simulink model "attitude3d"  (R2019b)
settings: Solver=ode4  StartTime=0.0  StopTime=6530  FixedStep=10  RelTol=1e-3
values from neighbouring files (symbols this model uses):
  P_E =     [P_E.mat]
  P_F =     [P_F.mat]
  P_X =     [P_X.mat]
undefined symbols (not defined in the file or in its folder): P
libraries: vrlib x14, simulink x5, dspstat3 x4, commfilt2 x2
(part 1 of 2)
settings Model: Creator=ggarrett  LastModifiedBy=ggarrett
settings DataIOCC: ExternalInput=x  LoadExternalInput=on  SaveFormat=Array  TimeSaveName=t  OutputSaveName=F
settings HardwareCC: TargetBitPerLong=64  TargetBitPerPointer=64  TargetBitPerSizeT=64  TargetBitPerPtrDiffT=64  TargetLongLongMode=on  TargetIntDivRoundTo=Zero  TargetEndianess=LittleEndian  TargetWordSize=64  TargetHWDeviceType=MATLAB Host  ProdEqTarget=off
settings RTWCC: Description=Rapid Simulation Target  SystemTargetFile=rsim.tlc  TemplateMakefile=rsim_default_tmf  RTWCompilerOptimization=on
settings RSimTargetCC: TargetLangStandard=C99 (ISO)  GeneratePreprocessorConditionals=Use local settings  PreserveStateflowLocalDataDimensions=off

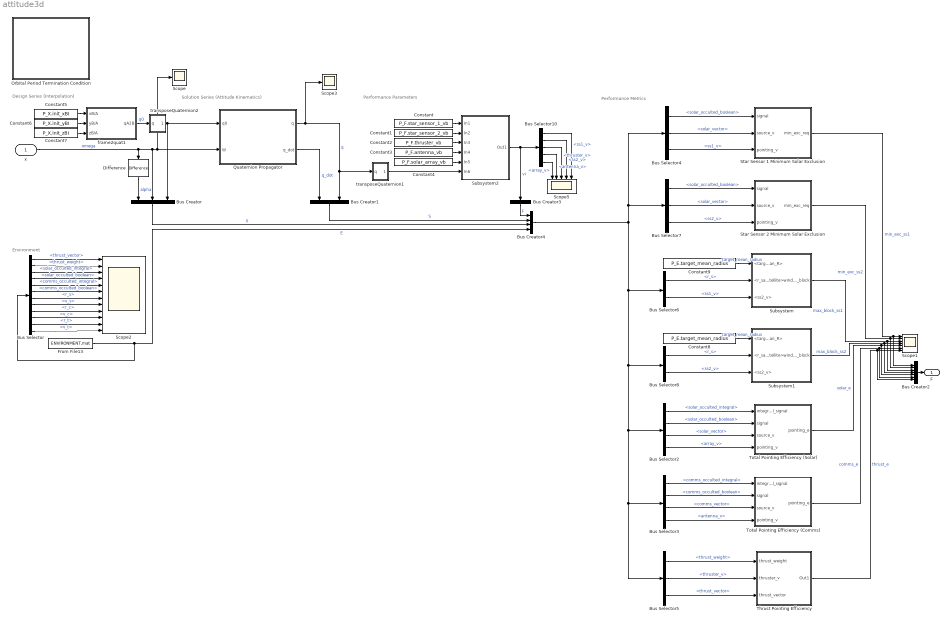
== system attitude3d ==
  note: Performance Metrics
  note: Solution Series (Attitude Kinematics)
  note: Design Series (Interpolation)
  note: Performance Parameters
  note: Environment
  x : Inport  OutDataTypeStr=double  PortDimensions=3
  Bus Creator : BusCreator  Inputs=3
  Bus Creator1 : BusCreator  Inputs=2
  Bus Creator2 : BusCreator  Inputs=7
  Bus Creator3 : BusCreator  Inputs=1
  Bus Creator4 : BusCreator  Inputs=4
  Bus Selector : BusSelector  OutputSignals=thrust_vector,thrust_weight,solar_occulted_integral,solar_occulted_boolean,comms_occulted_integral,comms_occulted_boolean,r_s,v_s,r_c,v_c,r_t,v_t
  Bus Selector10 : BusSelector  OutputSignals=ss1_v,ss2_v,thruster_v,antenna_v,array_v
  Bus Selector2 : BusSelector  OutputSignals=E.solar_occulted_integral,E.solar_occulted_boolean,E.solar_vector,F.vi.array_v
  Bus Selector3 : BusSelector  OutputSignals=E.comms_occulted_integral,E.comms_occulted_boolean,E.comms_vector,F.vi.antenna_v
  Bus Selector4 : BusSelector  OutputSignals=E.solar_occulted_boolean,E.solar_vector,F.vi.ss1_v
  Bus Selector5 : BusSelector  OutputSignals=E.thrust_weight,F.vi.thruster_v,E.thrust_vector
  Bus Selector6 : BusSelector  OutputSignals=E.r_s,F.vi.ss1_v
  Bus Selector7 : BusSelector  OutputSignals=E.solar_occulted_boolean,E.solar_vector,F.vi.ss2_v
  Bus Selector8 : BusSelector  OutputSignals=E.r_s,F.vi.ss2_v
  Constant : Constant  Value=P_F.star_sensor_1_vb
  Constant1 : Constant  Value=P_F.star_sensor_2_vb
  Constant2 : Constant  Value=P_F.thruster_vb
  Constant3 : Constant  Value=P_F.antenna_vb
  Constant4 : Constant  Value=P_F.solar_array_vb
  Constant5 : Constant  Value=P_X.init_xBI
  Constant6 : Constant  Value=P_X.init_yBI
  Constant7 : Constant  Value=P_X.init_zBI
  Constant8 : Constant  Value=P_E.target_mean_radius
  Constant9 : Constant  Value=P_E.target_mean_radius
  Difference : simulink/Discrete/Difference  ICPrevInput=0.0  OutMin=[]  OutMax=[]  OutDataType=fixdt(1, 16)  OutScaling=2^-10  DoSatur=off
  From File13 : FromFile  FileName=ENVIRONMENT.mat  OutDataTypeStr=Bus: ENVIRONMENT  SampleTime=0
  Orbital Period Termination Condition : Subsystem
  Quaternion Propagator : Subsystem
  Scope : Scope
  Scope1 : Scope  NumInputPorts=7
  Scope2 : Scope  NumInputPorts=12
  Scope3 : Scope
  Scope5 : Scope  NumInputPorts=5
  Star Sensor 1 Minimum Solar Exclusion : Subsystem
  Star Sensor 2 Minimum Solar Exclusion : Subsystem
  Subsystem : Subsystem
  Subsystem1 : Subsystem
  Subsystem2 : Subsystem
  Thrust Pointing Efficiency : Subsystem
  Total Pointing Efficiency (Comms) : Subsystem
  Total Pointing Efficiency (Solar) : Subsystem
  frame2quat1 : Subsystem  mask(Compute quaternion from 3 orthogonal unit vectors){Alabel=I, Blabel=B}
      mask prompts: Alabel "Label for origin frame"; Blabel "Label for target frame"
      mask help: Determines the attitude quaternion representing the rotation which transforms the origin frame into the target frame, from the unit vectors of target frame expressed in origin frame.
      mask Display:
      | port_label('input',1,['x',Blabel,'/',Alabel]);
      | port_label('input',2,['y',Blabel,'/',Alabel]);
      | port_label('input',3,['z',Blabel,'/',Alabel]);
      | port_label('output',1,['q',Alabel,'2',Blabel]);
  transposeQuaternion1 : Subsystem  mask(transposeQuaternion){}
      mask help:
      | Compute the transpose (inverse or conjugate) of the input quaternion
      |
      | Inputs:
      |   q     Quaternion
      |
      | Outputs:
      |   qt     Transpose of the input quaternion
      mask Help: eval('starDoc simulink/transposeQuaternion');
      mask Display: disp('q''');
  transposeQuaternion2 : Subsystem  mask(transposeQuaternion){}
      mask help:
      | Compute the transpose (inverse or conjugate) of the input quaternion
      |
      | Inputs:
      |   q     Quaternion
      |
      | Outputs:
      |   qt     Transpose of the input quaternion
      mask Help: eval('starDoc simulink/transposeQuaternion');
      mask Display: disp('q''');
  F : Outport  PortDimensions=7
  wires:
  x/1 -> Bus Creator/2, Scope/1, Quaternion Propagator/2(W), Difference/1  "omega"
  Difference/1 -> Bus Creator/1  "alpha"
  Quaternion Propagator/2(q_dot) -> Bus Creator1/1  "q_dot"
  Bus Creator/1 -> Bus Creator4/3  "X"
  Bus Creator1/1 -> Bus Creator4/2  "S"
  Quaternion Propagator/1(q) -> Scope3/1, Bus Creator1/2, transposeQuaternion1/1(q)  "q"
  Bus Creator3/1 -> Bus Creator4/1  "F"
  Bus Creator4/1 -> Bus Selector5/1, Bus Selector3/1, Bus Selector2/1, Bus Selector8/1, Bus Selector6/1, Bus Selector4/1, Bus Selector7/1
  Bus Selector2/3 -> Total Pointing Efficiency (Solar)/3(source_v)  "<solar_vector>"
  Bus Selector2/4 -> Total Pointing Efficiency (Solar)/4(pointing_v)  "<array_v>"
  Bus Selector2/1 -> Total Pointing Efficiency (Solar)/1(integral_signal)  "<solar_occulted_integral>"
  Bus Selector2/2 -> Total Pointing Efficiency (Solar)/2(signal)  "<solar_occulted_boolean>"
  Bus Selector3/4 -> Total Pointing Efficiency (Comms)/4(pointing_v)  "<antenna_v>"
  Bus Selector3/1 -> Total Pointing Efficiency (Comms)/1(integral_signal)  "<comms_occulted_integral>"
  Bus Selector3/3 -> Total Pointing Efficiency (Comms)/3(source_v)  "<comms_vector>"
  Bus Selector3/2 -> Total Pointing Efficiency (Comms)/2(signal)  "<comms_occulted_boolean>"
  Bus Selector4/3 -> Star Sensor 1 Minimum Solar Exclusion/3(pointing_v)  "<ss1_v>"
  Bus Selector4/1 -> Star Sensor 1 Minimum Solar Exclusion/1(signal)  "<solar_occulted_boolean>"
  Bus Selector4/2 -> Star Sensor 1 Minimum Solar Exclusion/2(source_v)  "<solar_vector>"
  Bus Selector5/3 -> Thrust Pointing Efficiency/3(thrust_vector)  "<thrust_vector>"
  Bus Selector7/3 -> Star Sensor 2 Minimum Solar Exclusion/3(pointing_v)  "<ss2_v>"
  Bus Selector7/1 -> Star Sensor 2 Minimum Solar Exclusion/1(signal)  "<solar_occulted_boolean>"
  Bus Selector7/2 -> Star Sensor 2 Minimum Solar Exclusion/2(source_v)  "<solar_vector>"
  Subsystem1/1(window_block) -> Bus Creator2/4, Scope1/4  "max_block_ss2"
  Subsystem/1(window_block) -> Bus Creator2/3, Scope1/3  "max_block_ss1"
  Star Sensor 2 Minimum Solar Exclusion/1(min_exc_req) -> Bus Creator2/2, Scope1/2  "min_exc_ss2"
  Star Sensor 1 Minimum Solar Exclusion/1(min_exc_req) -> Bus Creator2/1, Scope1/1  "min_exc_ss1"
  Total Pointing Efficiency (Solar)/1(pointing_e) -> Bus Creator2/5, Scope1/5  "solar_e"
  Total Pointing Efficiency (Comms)/1(pointing_e) -> Bus Creator2/6, Scope1/6  "comms_e"
  Thrust Pointing Efficiency/1(Out1) -> Bus Creator2/7, Scope1/7  "thrust_e"
  From File13/1 -> Bus Selector/1, Bus Creator4/4  "E"
  Bus Selector/1 -> Scope2/1  "<thrust_vector>"
  Bus Selector/2 -> Scope2/2  "<thrust_weight>"
  Bus Selector/3 -> Scope2/3  "<solar_occulted_integral>"
  Bus Selector/12 -> Scope2/12  "<v_t>"
  Bus Selector/11 -> Scope2/11  "<r_t>"
  Bus Selector/10 -> Scope2/10  "<v_c>"
  Bus Selector/9 -> Scope2/9  "<r_c>"
  Bus Selector/8 -> Scope2/8  "<v_s>"
  Bus Selector/7 -> Scope2/7  "<r_s>"
  Bus Selector/6 -> Scope2/6  "<comms_occulted_boolean>"
  Bus Selector/5 -> Scope2/5  "<comms_occulted_integral>"
  Bus Selector/4 -> Scope2/4  "<solar_occulted_boolean>"
  Constant5/1 -> frame2quat1/1(xB/A)
  Constant6/1 -> frame2quat1/2(yB/A)
  Bus Selector10/5 -> Scope5/1  "<array_v>"
  Bus Selector10/4 -> Scope5/2  "<antenna_v>"
  Bus Selector10/3 -> Scope5/3  "<thruster_v>"
  Bus Selector10/2 -> Scope5/4  "<ss2_v>"
  Bus Selector10/1 -> Scope5/5  "<ss1_v>"
  Subsystem2/1(Out1) -> Bus Creator3/1, Bus Selector10/1  "vi"
  Constant7/1 -> frame2quat1/3(zB/A)
  Constant/1 -> Subsystem2/1(In1)
  Constant1/1 -> Subsystem2/2(In2)
  Constant2/1 -> Subsystem2/3(In3)
  Constant3/1 -> Subsystem2/4(In4)
  Constant4/1 -> Subsystem2/5(In5)
  transposeQuaternion1/1(q') -> Subsystem2/6(In6)
  Bus Selector8/1 -> Subsystem1/2(<r_satellite>)  "<r_s>"
  Bus Selector8/2 -> Subsystem1/3(<ss2_v>)  "<ss2_v>"
  Constant8/1 -> Subsystem1/1(<target_mean_R>)  "target_mean_radius"
  Bus Selector6/2 -> Subsystem/3(<ss2_v>)  "<ss1_v>"
  Bus Selector6/1 -> Subsystem/2(<r_satellite>)  "<r_s>"
  Constant9/1 -> Subsystem/1(<target_mean_R>)  "target_mean_radius"
  Bus Selector5/1 -> Thrust Pointing Efficiency/1(thrust_weight)  "<thrust_weight>"
  Bus Selector5/2 -> Thrust Pointing Efficiency/2(thruster_v)  "<thruster_v>"
  frame2quat1/1(qA2B) -> transposeQuaternion2/1(q)  "q0"
  transposeQuaternion2/1(q') -> Bus Creator/3, Quaternion Propagator/1(q0)
  Bus Creator2/1 -> F/1

== system attitude3d/Orbital Period Termination Condition ==
  Clock1 : Clock
  Compare To Zero : simulink/Logic and Bit Operations/Compare To Zero  relop=<=  OutDataTypeStr=boolean
  Constant : Constant  Value=0.999*P_E.P
  Scope : Scope  NumInputPorts=2
  Stop Simulation : Stop
  Sum : Sum  Inputs=|-+
  wires:
  Constant/1 -> Scope/1, Sum/2
  Clock1/1 -> Scope/2, Sum/1
  Sum/1 -> Compare To Zero/1
  Compare To Zero/1 -> Stop Simulation/1

== system attitude3d/Quaternion Propagator ==
  q0 : Inport
  W : Inport  Port=2
  Integrator : Integrator  InitialConditionSource=external
  Quaternion Normed : MATLAB Function  TreatAsAtomicUnit=on
  qDot : Subsystem  Tag=40  mask(W2dqdt){}
      mask help:
      | Compute quaternion derivative from instantaneous angular velocity of the rigid body expressed in body frame :
      | dq/dt = 0.5*q*W
      | K. Lagadec 1998
  q : Outport
  q_dot : Outport  Port=2
  wires:
  Integrator/1 -> Quaternion Normed/1(u)
  q0/1 -> Integrator/2
  Quaternion Normed/1(y) -> qDot/1(q), q/1
  W/1 -> qDot/2(W)
  qDot/1(qDot) -> Integrator/1, q_dot/1

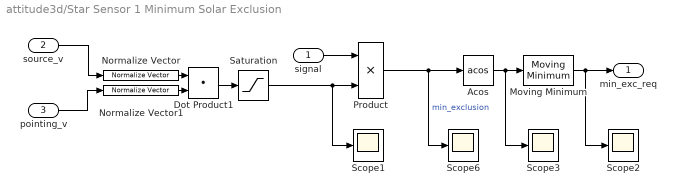
== system attitude3d/Star Sensor 1 Minimum Solar Exclusion ==
  signal : Inport
  source_v : Inport  Port=2
  pointing_v : Inport  Port=3
  Acos : Trigonometry  Operator=acos
  Dot Product1 : DotProduct  InputSameDT=on  OutDataTypeStr=Inherit: Inherit via internal rule
  Moving Minimum : dspstat3/Moving Minimum  SpecifyWindowLength=off  WindowLength=int16(P/10)  SimulateUsing=Code generation
      settings: SourceProductName=DSP System Toolbox  SourceProductBaseCode=DS
  Normalize Vector : vrlib/Utilities/Normalize Vector  maxzero=0
      settings: SourceProductName=Simulink
  Normalize Vector1 : vrlib/Utilities/Normalize Vector  maxzero=0
      settings: SourceProductName=Simulink
  Product : Product
  Saturation : Saturate  UpperLimit=1.0  LowerLimit=0
  Scope{1..3,6} (4 alike) : Scope
  min_exc_req : Outport
  wires:
  Dot Product1/1 -> Saturation/1
  Normalize Vector1/1 -> Dot Product1/2
  signal/1 -> Product/1
  source_v/1 -> Normalize Vector/1
  pointing_v/1 -> Normalize Vector1/1
  Normalize Vector/1 -> Dot Product1/1
  Saturation/1 -> Scope1/1, Product/2
  Product/1 -> Scope6/1, Acos/1  "min_exclusion"
  Acos/1 -> Scope3/1, Moving Minimum/1
  Moving Minimum/1 -> Scope2/1, min_exc_req/1

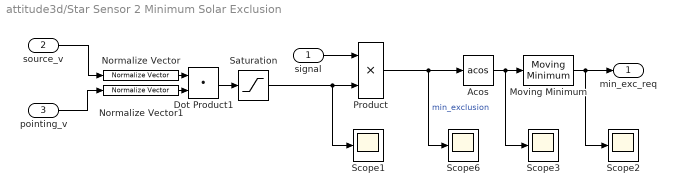
== system attitude3d/Star Sensor 2 Minimum Solar Exclusion ==
  signal : Inport
  source_v : Inport  Port=2
  pointing_v : Inport  Port=3
  Acos : Trigonometry  Operator=acos
  Dot Product1 : DotProduct  InputSameDT=on  OutDataTypeStr=Inherit: Inherit via internal rule
  Moving Minimum : dspstat3/Moving Minimum  SpecifyWindowLength=off  WindowLength=int16(P/10)  SimulateUsing=Code generation
      settings: SourceProductName=DSP System Toolbox  SourceProductBaseCode=DS
  Normalize Vector : vrlib/Utilities/Normalize Vector  maxzero=0
      settings: SourceProductName=Simulink
  Normalize Vector1 : vrlib/Utilities/Normalize Vector  maxzero=0
      settings: SourceProductName=Simulink
  Product : Product
  Saturation : Saturate  UpperLimit=1.0  LowerLimit=0
  Scope{1..3,6} (4 alike) : Scope
  min_exc_req : Outport
  wires:
  Dot Product1/1 -> Saturation/1
  Normalize Vector1/1 -> Dot Product1/2
  signal/1 -> Product/1
  source_v/1 -> Normalize Vector/1
  pointing_v/1 -> Normalize Vector1/1
  Normalize Vector/1 -> Dot Product1/1
  Saturation/1 -> Scope1/1, Product/2
  Product/1 -> Scope6/1, Acos/1  "min_exclusion"
  Acos/1 -> Scope3/1, Moving Minimum/1
  Moving Minimum/1 -> Scope2/1, min_exc_req/1

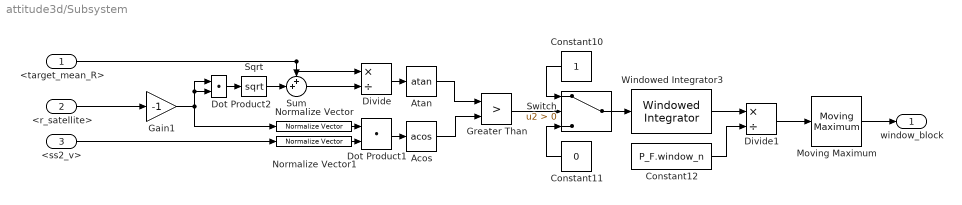
== system attitude3d/Subsystem ==
  <target_mean_R> : Inport
  <r_satellite> : Inport  Port=2
  <ss2_v> : Inport  Port=3
  Acos : Trigonometry  Operator=acos
  Atan : Trigonometry  Operator=atan
  Constant10 : Constant
  Constant11 : Constant  Value=0
  Constant12 : Constant  Value=P_F.window_n
  Divide : Product  Inputs=*/
  Divide1 : Product  Inputs=*/
  Dot Product1 : DotProduct  InputSameDT=on  OutDataTypeStr=Inherit: Inherit via internal rule
  Dot Product2 : DotProduct  InputSameDT=on  OutDataTypeStr=Inherit: Inherit via internal rule
  Gain1 : Gain  Gain=-1
  Greater Than : RelationalOperator  Operator=>  OutDataTypeStr=boolean  RndMeth=Simplest
  Moving Maximum : dspstat3/Moving Maximum  SpecifyWindowLength=off  WindowLength=4  SimulateUsing=Code generation
      settings: SourceProductName=DSP System Toolbox  SourceProductBaseCode=DS
  Normalize Vector : vrlib/Utilities/Normalize Vector  maxzero=0
      settings: SourceProductName=Simulink
  Normalize Vector1 : vrlib/Utilities/Normalize Vector  maxzero=0
      settings: SourceProductName=Simulink
  Sqrt : Sqrt  SaturateOnIntegerOverflow=on
  Sum : Sum  Inputs=++|
  Switch : Switch  Criteria=u2 > Threshold
  Windowed Integrator3 : commfilt2/Windowed Integrator  integperiod=P_F.window_n  InputProcessing=Columns as channels (frame based)  roundingMode=Floor  overflowMode=off  coeffDataTypeStr=Inherit: Same word length as input  coeffMin=[]  coeffMax=[]  coeffLastDataTypeStr=Inherit: Same word length as input  accumDataTypeStr=Inherit: Same as product output  accumLastDataTypeStr=Inherit: Same as product output  outputDataTypeStr=Inherit: Same as accumulator  outputMin=[]  outputMax=[]  outputLastDataTypeStr=Inherit: Same as accumulator
      settings: SourceProductName=Communications Toolbox  SourceProductBaseCode=CM
  window_block : Outport
  wires:
  Sum/1 -> Divide/2
  Dot Product1/1 -> Acos/1
  Normalize Vector/1 -> Dot Product1/1
  Divide1/1 -> Moving Maximum/1
  Constant12/1 -> Divide1/2
  Divide/1 -> Atan/1
  Atan/1 -> Greater Than/1
  Dot Product2/1 -> Sqrt/1
  Moving Maximum/1 -> window_block/1
  Acos/1 -> Greater Than/2
  <r_satellite>/1 -> Gain1/1
  <ss2_v>/1 -> Normalize Vector1/1
  Normalize Vector1/1 -> Dot Product1/2
  Sqrt/1 -> Sum/2
  Constant11/1 -> Switch/3
  Constant10/1 -> Switch/1
  Greater Than/1 -> Switch/2
  <target_mean_R>/1 -> Divide/1, Sum/1
  Gain1/1 -> Normalize Vector/1, Dot Product2/1, Dot Product2/2
  Windowed Integrator3/1 -> Divide1/1
  Switch/1 -> Windowed Integrator3/1

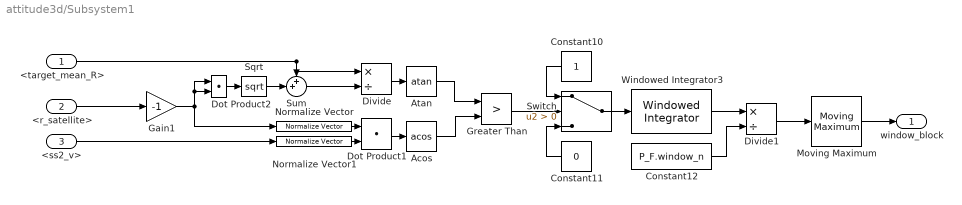
== system attitude3d/Subsystem1 ==
  <target_mean_R> : Inport
  <r_satellite> : Inport  Port=2
  <ss2_v> : Inport  Port=3
  Acos : Trigonometry  Operator=acos
  Atan : Trigonometry  Operator=atan
  Constant10 : Constant
  Constant11 : Constant  Value=0
  Constant12 : Constant  Value=P_F.window_n
  Divide : Product  Inputs=*/
  Divide1 : Product  Inputs=*/
  Dot Product1 : DotProduct  InputSameDT=on  OutDataTypeStr=Inherit: Inherit via internal rule
  Dot Product2 : DotProduct  InputSameDT=on  OutDataTypeStr=Inherit: Inherit via internal rule
  Gain1 : Gain  Gain=-1
  Greater Than : RelationalOperator  Operator=>  OutDataTypeStr=boolean  RndMeth=Simplest
  Moving Maximum : dspstat3/Moving Maximum  SpecifyWindowLength=off  WindowLength=4  SimulateUsing=Code generation
      settings: SourceProductName=DSP System Toolbox  SourceProductBaseCode=DS
  Normalize Vector : vrlib/Utilities/Normalize Vector  maxzero=0
      settings: SourceProductName=Simulink
  Normalize Vector1 : vrlib/Utilities/Normalize Vector  maxzero=0
      settings: SourceProductName=Simulink
  Sqrt : Sqrt  SaturateOnIntegerOverflow=on
  Sum : Sum  Inputs=++|
  Switch : Switch  Criteria=u2 > Threshold
  Windowed Integrator3 : commfilt2/Windowed Integrator  integperiod=P_F.window_n  InputProcessing=Columns as channels (frame based)  roundingMode=Floor  overflowMode=off  coeffDataTypeStr=Inherit: Same word length as input  coeffMin=[]  coeffMax=[]  coeffLastDataTypeStr=Inherit: Same word length as input  accumDataTypeStr=Inherit: Same as product output  accumLastDataTypeStr=Inherit: Same as product output  outputDataTypeStr=Inherit: Same as accumulator  outputMin=[]  outputMax=[]  outputLastDataTypeStr=Inherit: Same as accumulator
      settings: SourceProductName=Communications Toolbox  SourceProductBaseCode=CM
  window_block : Outport
  wires:
  Sum/1 -> Divide/2
  Dot Product1/1 -> Acos/1
  Normalize Vector/1 -> Dot Product1/1
  Divide1/1 -> Moving Maximum/1
  Constant12/1 -> Divide1/2
  Divide/1 -> Atan/1
  Atan/1 -> Greater Than/1
  Dot Product2/1 -> Sqrt/1
  Moving Maximum/1 -> window_block/1
  Acos/1 -> Greater Than/2
  <r_satellite>/1 -> Gain1/1
  <ss2_v>/1 -> Normalize Vector1/1
  Normalize Vector1/1 -> Dot Product1/2
  Sqrt/1 -> Sum/2
  Constant11/1 -> Switch/3
  Constant10/1 -> Switch/1
  Greater Than/1 -> Switch/2
  <target_mean_R>/1 -> Divide/1, Sum/1
  Gain1/1 -> Normalize Vector/1, Dot Product2/1, Dot Product2/2
  Windowed Integrator3/1 -> Divide1/1
  Switch/1 -> Windowed Integrator3/1

== system attitude3d/Subsystem2 ==
  In1 : Inport
  In2 : Inport  Port=2
  In3 : Inport  Port=3
  In4 : Inport  Port=4
  In5 : Inport  Port=5
  In6 : Inport  Port=6
  Bus Creator2 : BusCreator  Inputs=5
  frame change5 : Subsystem  mask(Frame change){inLabel=b, outLabel=i}
      mask prompts: inLabel "Label for initial frame"; outLabel "Label for target frame"
      mask help: Express input vector in frame B, using the quaternion describing the rotation from frame A to frame B.
      mask Display:
      | port_label('input',1,['v',inLabel]);
      | port_label('output',1,['v',outLabel]);
      | port_label('input',2,['q',inLabel,'2',outLabel]);
  frame change6 : Subsystem  mask(Frame change){inLabel=b, outLabel=i}
      mask prompts: inLabel "Label for initial frame"; outLabel "Label for target frame"
      mask help: Express input vector in frame B, using the quaternion describing the rotation from frame A to frame B.
      mask Display:
      | port_label('input',1,['v',inLabel]);
      | port_label('output',1,['v',outLabel]);
      | port_label('input',2,['q',inLabel,'2',outLabel]);
  frame change7 : Subsystem  mask(Frame change){inLabel=b, outLabel=i}
      mask prompts: inLabel "Label for initial frame"; outLabel "Label for target frame"
      mask help: Express input vector in frame B, using the quaternion describing the rotation from frame A to frame B.
      mask Display:
      | port_label('input',1,['v',inLabel]);
      | port_label('output',1,['v',outLabel]);
      | port_label('input',2,['q',inLabel,'2',outLabel]);
  frame change8 : Subsystem  mask(Frame change){inLabel=b, outLabel=i}
      mask prompts: inLabel "Label for initial frame"; outLabel "Label for target frame"
      mask help: Express input vector in frame B, using the quaternion describing the rotation from frame A to frame B.
      mask Display:
      | port_label('input',1,['v',inLabel]);
      | port_label('output',1,['v',outLabel]);
      | port_label('input',2,['q',inLabel,'2',outLabel]);
  frame change9 : Subsystem  mask(Frame change){inLabel=b, outLabel=i}
      mask prompts: inLabel "Label for initial frame"; outLabel "Label for target frame"
      mask help: Express input vector in frame B, using the quaternion describing the rotation from frame A to frame B.
      mask Display:
      | port_label('input',1,['v',inLabel]);
      | port_label('output',1,['v',outLabel]);
      | port_label('input',2,['q',inLabel,'2',outLabel]);
  Out1 : Outport
  wires:
  Bus Creator2/1 -> Out1/1
  frame change5/1(vB) -> Bus Creator2/1  "ss1_v"
  In5/1 -> frame change9/1(vA)
  In3/1 -> frame change7/1(vA)
  In4/1 -> frame change8/1(vA)
  In1/1 -> frame change5/1(vA)
  frame change6/1(vB) -> Bus Creator2/2  "ss2_v"
  In6/1 -> frame change9/2(qA2B), frame change8/2(qA2B), frame change7/2(qA2B), frame change6/2(qA2B), frame change5/2(qA2B)
  frame change8/1(vB) -> Bus Creator2/4  "antenna_v"
  frame change9/1(vB) -> Bus Creator2/5  "array_v"
  frame change7/1(vB) -> Bus Creator2/3  "thruster_v"
  In2/1 -> frame change6/1(vA)

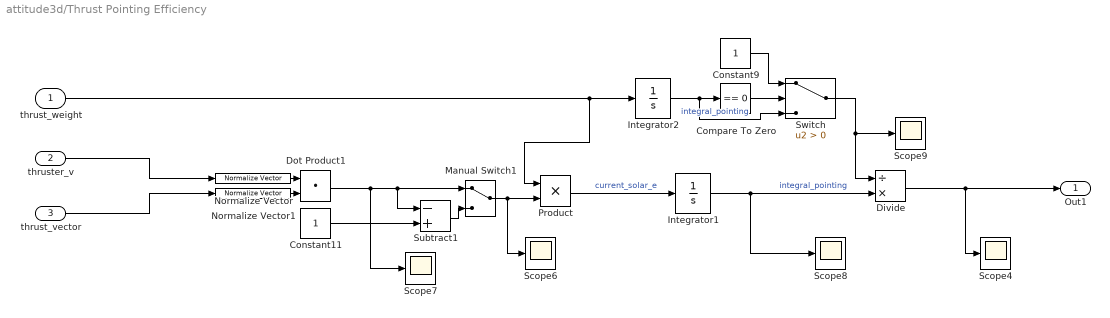
== system attitude3d/Thrust Pointing Efficiency ==
  thrust_weight : Inport
  thruster_v : Inport  Port=2
  thrust_vector : Inport  Port=3
  Compare To Zero : simulink/Logic and Bit Operations/Compare To Zero  relop===  OutDataTypeStr=boolean
  Constant11 : Constant
  Constant9 : Constant
  Divide : Product  Inputs=/*
  Dot Product1 : DotProduct  InputSameDT=on  OutDataTypeStr=Inherit: Inherit via internal rule
  Integrator1 : Integrator
  Integrator2 : Integrator
  Manual Switch1 : ManualSwitch
  Normalize Vector : vrlib/Utilities/Normalize Vector  maxzero=0
      settings: SourceProductName=Simulink
  Normalize Vector1 : vrlib/Utilities/Normalize Vector  maxzero=0
      settings: SourceProductName=Simulink
  Product : Product
  Scope{4,6..9} (5 alike) : Scope
  Subtract1 : Sum  Inputs=-+
  Switch : Switch  Criteria=u2 > Threshold
  Out1 : Outport
  wires:
  Constant9/1 -> Switch/1
  Normalize Vector/1 -> Dot Product1/1
  Product/1 -> Integrator1/1  "current_solar_e"
  Manual Switch1/1 -> Scope6/1, Product/2
  Dot Product1/1 -> Scope7/1, Subtract1/1, Manual Switch1/1
  Integrator1/1 -> Scope8/1, Divide/2  "integral_pointing"
  Switch/1 -> Scope9/1, Divide/1
  Integrator2/1 -> Switch/3, Compare To Zero/1  "integral_pointing"
  Normalize Vector1/1 -> Dot Product1/2
  Constant11/1 -> Subtract1/2
  Divide/1 -> Out1/1, Scope4/1
  Subtract1/1 -> Manual Switch1/2
  thrust_vector/1 -> Normalize Vector1/1
  Compare To Zero/1 -> Switch/2
  thrust_weight/1 -> Product/1, Integrator2/1
  thruster_v/1 -> Normalize Vector/1

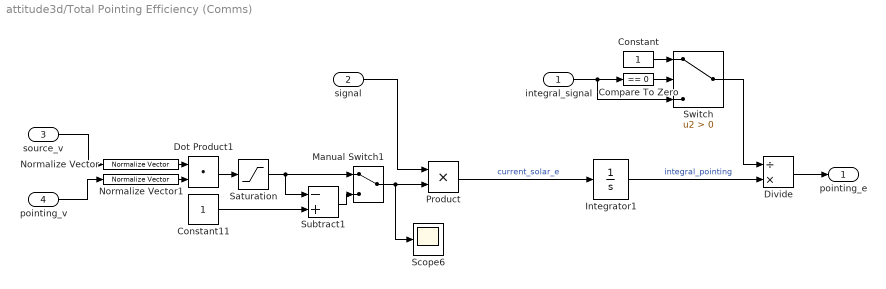
== system attitude3d/Total Pointing Efficiency (Comms) ==
  integral_signal : Inport
  signal : Inport  Port=2
  source_v : Inport  Port=3
  pointing_v : Inport  Port=4
  Compare To Zero : simulink/Logic and Bit Operations/Compare To Zero  relop===  OutDataTypeStr=boolean
  Constant : Constant
  Constant11 : Constant
  Divide : Product  Inputs=/*
  Dot Product1 : DotProduct  InputSameDT=on  OutDataTypeStr=Inherit: Inherit via internal rule
  Integrator1 : Integrator
  Manual Switch1 : ManualSwitch
  Normalize Vector : vrlib/Utilities/Normalize Vector  maxzero=0
      settings: SourceProductName=Simulink
  Normalize Vector1 : vrlib/Utilities/Normalize Vector  maxzero=0
      settings: SourceProductName=Simulink
  Product : Product
  Saturation : Saturate  UpperLimit=1.0  LowerLimit=0
  Scope6 : Scope
  Subtract1 : Sum  Inputs=-+
  Switch : Switch  Criteria=u2 > Threshold
  pointing_e : Outport
  wires:
  Subtract1/1 -> Manual Switch1/2
  Dot Product1/1 -> Saturation/1
  Normalize Vector1/1 -> Dot Product1/2
  Saturation/1 -> Subtract1/1, Manual Switch1/1
  Product/1 -> Integrator1/1  "current_solar_e"
  integral_signal/1 -> Compare To Zero/1, Switch/3
  signal/1 -> Product/1
  source_v/1 -> Normalize Vector/1
  Constant11/1 -> Subtract1/2
  Manual Switch1/1 -> Scope6/1, Product/2
  Divide/1 -> pointing_e/1
  pointing_v/1 -> Normalize Vector1/1
  Integrator1/1 -> Divide/2  "integral_pointing"
  Normalize Vector/1 -> Dot Product1/1
  Compare To Zero/1 -> Switch/2
  Constant/1 -> Switch/1
  Switch/1 -> Divide/1

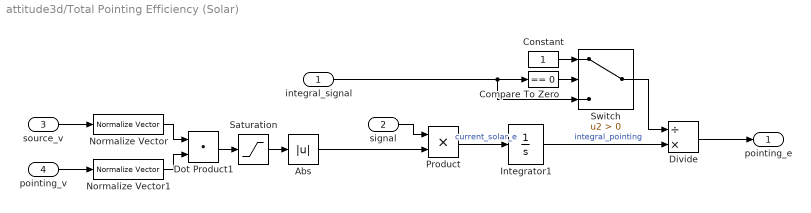
== system attitude3d/Total Pointing Efficiency (Solar) ==
  integral_signal : Inport
  signal : Inport  Port=2
  source_v : Inport  Port=3
  pointing_v : Inport  Port=4
  Abs : Abs
  Compare To Zero : simulink/Logic and Bit Operations/Compare To Zero  relop===  OutDataTypeStr=boolean
  Constant : Constant
  Divide : Product  Inputs=/*
  Dot Product1 : DotProduct  InputSameDT=on  OutDataTypeStr=Inherit: Inherit via internal rule
  Integrator1 : Integrator
  Normalize Vector : vrlib/Utilities/Normalize Vector  maxzero=0
      settings: SourceProductName=Simulink
  Normalize Vector1 : vrlib/Utilities/Normalize Vector  maxzero=0
      settings: SourceProductName=Simulink
  Product : Product
  Saturation : Saturate  UpperLimit=1.0  LowerLimit=-1.0
  Switch : Switch  Criteria=u2 > Threshold
  pointing_e : Outport
  wires:
  Dot Product1/1 -> Saturation/1
  Normalize Vector1/1 -> Dot Product1/2
  Product/1 -> Integrator1/1  "current_solar_e"
  integral_signal/1 -> Switch/3, Compare To Zero/1
  signal/1 -> Product/1
  source_v/1 -> Normalize Vector/1
  Divide/1 -> pointing_e/1
  pointing_v/1 -> Normalize Vector1/1
  Integrator1/1 -> Divide/2  "integral_pointing"
  Normalize Vector/1 -> Dot Product1/1
  Compare To Zero/1 -> Switch/2
  Constant/1 -> Switch/1
  Switch/1 -> Divide/1
  Saturation/1 -> Abs/1
  Abs/1 -> Product/2

== system attitude3d/frame2quat1 ==
  xB/A : Inport  PortDimensions=3
  yB/A : Inport  Port=2  PortDimensions=3
  zB/A : Inport  Port=3  PortDimensions=3
  MATLAB Function : MATLAB Function  TreatAsAtomicUnit=on
  qA2B : Outport  PortDimensions=4
  wires:
  xB/A/1 -> MATLAB Function/1(xB)
  yB/A/1 -> MATLAB Function/2(yB)
  zB/A/1 -> MATLAB Function/3(zB)
  MATLAB Function/1(qA2B) -> qA2B/1

== system attitude3d/transposeQuaternion1 ==
  q : Inport  PortDimensions=4
  Gain1 : Gain  Gain=[1 -1 -1 -1]  SaturateOnIntegerOverflow=on  OutDataTypeStr=Inherit: Same as input  ParamDataTypeStr=Inherit: Same as input
  q' : Outport  PortDimensions=4
  wires:
  q/1 -> Gain1/1
  Gain1/1 -> q'/1

== system attitude3d/transposeQuaternion2 ==
  q : Inport  PortDimensions=4
  Gain1 : Gain  Gain=[1 -1 -1 -1]  SaturateOnIntegerOverflow=on  OutDataTypeStr=Inherit: Same as input  ParamDataTypeStr=Inherit: Same as input
  q' : Outport  PortDimensions=4
  wires:
  q/1 -> Gain1/1
  Gain1/1 -> q'/1

== system attitude3d/Quaternion Propagator/qDot ==
  note: q_dot = 1/2 q.W
  q : Inport  PortDimensions=4
  W : Inport  Port=2  PortDimensions=3
  Constant : Constant  Value=0
  Gain : Gain  Gain=1/2  SaturateOnIntegerOverflow=on  OutDataTypeStr=Inherit: Same as input  ParamDataTypeStr=Inherit: Same as input
  Transform into quaternion : Mux  Inputs=2
  quat product : Subsystem
      mask Display:
      | plot(0.5+cos(linspace(0,2*pi,65))*0.3,0.5+sin(linspace(0,2*pi,65))*0.3);
      | plot([.29 .71],[.29 .71]);
      | plot([.71 .29],[.29 .71]);
  qDot : Outport  PortDimensions=4  InitialOutput=0
  wires:
  Constant/1 -> Transform into quaternion/1
  W/1 -> Transform into quaternion/2
  Transform into quaternion/1 -> quat product/2(q2)
  quat product/1(q1*q2) -> Gain/1
  Gain/1 -> qDot/1  "q_dot"
  q/1 -> quat product/1(q1)

== system attitude3d/Subsystem2/frame change5 ==
  vA : Inport
  qA2B : Inport  Port=2
  Constant : Constant
  Demux : Demux  Outputs=[1 3]
  Mux : Mux  Inputs=2
  Product : Product  Inputs=/*  SaturateOnIntegerOverflow=on  OutDataTypeStr=Inherit: Same as first input
  quat product : Subsystem
      mask Display:
      | plot(0.5+cos(linspace(0,2*pi,65))*0.3,0.5+sin(linspace(0,2*pi,65))*0.3);
      | plot([.29 .71],[.29 .71]);
      | plot([.71 .29],[.29 .71]);
  quat product1 : Subsystem
      mask Display:
      | plot(0.5+cos(linspace(0,2*pi,65))*0.3,0.5+sin(linspace(0,2*pi,65))*0.3);
      | plot([.29 .71],[.29 .71]);
      | plot([.71 .29],[.29 .71]);
  transposeQuaternion : Subsystem  mask(transposeQuaternion){}
      mask help:
      | Compute the transpose (inverse or conjugate) of the input quaternion
      |
      | Inputs:
      |   q     Quaternion
      |
      | Outputs:
      |   qt     Transpose of the input quaternion
      mask Help: eval('starDoc simulink/transposeQuaternion');
      mask Display: disp('q''');
  vB : Outport
  wires:
  Product/1 -> vB/1
  quat product1/1(q1*q2) -> Demux/1
  quat product/1(q1*q2) -> quat product1/1(q1)
  Mux/1 -> quat product/2(q2)
  transposeQuaternion/1(q') -> quat product/1(q1)
  qA2B/1 -> quat product1/2(q2), transposeQuaternion/1(q)
  vA/1 -> Mux/2
  Constant/1 -> Mux/1
  Demux/1 -> Product/1
  Demux/2 -> Product/2

== system attitude3d/Subsystem2/frame change6 ==
  vA : Inport
  qA2B : Inport  Port=2
  Constant : Constant
  Demux : Demux  Outputs=[1 3]
  Mux : Mux  Inputs=2
  Product : Product  Inputs=/*  SaturateOnIntegerOverflow=on  OutDataTypeStr=Inherit: Same as first input
  quat product : Subsystem
      mask Display:
      | plot(0.5+cos(linspace(0,2*pi,65))*0.3,0.5+sin(linspace(0,2*pi,65))*0.3);
      | plot([.29 .71],[.29 .71]);
      | plot([.71 .29],[.29 .71]);
  quat product1 : Subsystem
      mask Display:
      | plot(0.5+cos(linspace(0,2*pi,65))*0.3,0.5+sin(linspace(0,2*pi,65))*0.3);
      | plot([.29 .71],[.29 .71]);
      | plot([.71 .29],[.29 .71]);
  transposeQuaternion : Subsystem  mask(transposeQuaternion){}
      mask help:
      | Compute the transpose (inverse or conjugate) of the input quaternion
      |
      | Inputs:
      |   q     Quaternion
      |
      | Outputs:
      |   qt     Transpose of the input quaternion
      mask Help: eval('starDoc simulink/transposeQuaternion');
      mask Display: disp('q''');
  vB : Outport
  wires:
  Product/1 -> vB/1
  quat product1/1(q1*q2) -> Demux/1
  quat product/1(q1*q2) -> quat product1/1(q1)
  Mux/1 -> quat product/2(q2)
  transposeQuaternion/1(q') -> quat product/1(q1)
  qA2B/1 -> quat product1/2(q2), transposeQuaternion/1(q)
  vA/1 -> Mux/2
  Constant/1 -> Mux/1
  Demux/1 -> Product/1
  Demux/2 -> Product/2

== system attitude3d/Subsystem2/frame change7 ==
  vA : Inport
  qA2B : Inport  Port=2
  Constant : Constant
  Demux : Demux  Outputs=[1 3]
  Mux : Mux  Inputs=2
  Product : Product  Inputs=/*  SaturateOnIntegerOverflow=on  OutDataTypeStr=Inherit: Same as first input
  quat product : Subsystem
      mask Display:
      | plot(0.5+cos(linspace(0,2*pi,65))*0.3,0.5+sin(linspace(0,2*pi,65))*0.3);
      | plot([.29 .71],[.29 .71]);
      | plot([.71 .29],[.29 .71]);
  quat product1 : Subsystem
      mask Display:
      | plot(0.5+cos(linspace(0,2*pi,65))*0.3,0.5+sin(linspace(0,2*pi,65))*0.3);
      | plot([.29 .71],[.29 .71]);
      | plot([.71 .29],[.29 .71]);
  transposeQuaternion : Subsystem  mask(transposeQuaternion){}
      mask help:
      | Compute the transpose (inverse or conjugate) of the input quaternion
      |
      | Inputs:
      |   q     Quaternion
      |
      | Outputs:
      |   qt     Transpose of the input quaternion
      mask Help: eval('starDoc simulink/transposeQuaternion');
      mask Display: disp('q''');
  vB : Outport
  wires:
  Product/1 -> vB/1
  quat product1/1(q1*q2) -> Demux/1
  quat product/1(q1*q2) -> quat product1/1(q1)
  Mux/1 -> quat product/2(q2)
  transposeQuaternion/1(q') -> quat product/1(q1)
  qA2B/1 -> quat product1/2(q2), transposeQuaternion/1(q)
  vA/1 -> Mux/2
  Constant/1 -> Mux/1
  Demux/1 -> Product/1
  Demux/2 -> Product/2

== system attitude3d/Subsystem2/frame change8 ==
  vA : Inport
  qA2B : Inport  Port=2
  Constant : Constant
  Demux : Demux  Outputs=[1 3]
  Mux : Mux  Inputs=2
  Product : Product  Inputs=/*  SaturateOnIntegerOverflow=on  OutDataTypeStr=Inherit: Same as first input
  quat product : Subsystem
      mask Display:
      | plot(0.5+cos(linspace(0,2*pi,65))*0.3,0.5+sin(linspace(0,2*pi,65))*0.3);
      | plot([.29 .71],[.29 .71]);
      | plot([.71 .29],[.29 .71]);
  quat product1 : Subsystem
      mask Display:
      | plot(0.5+cos(linspace(0,2*pi,65))*0.3,0.5+sin(linspace(0,2*pi,65))*0.3);
      | plot([.29 .71],[.29 .71]);
      | plot([.71 .29],[.29 .71]);
  transposeQuaternion : Subsystem  mask(transposeQuaternion){}
      mask help:
      | Compute the transpose (inverse or conjugate) of the input quaternion
      |
      | Inputs:
      |   q     Quaternion
      |
      | Outputs:
      |   qt     Transpose of the input quaternion
      mask Help: eval('starDoc simulink/transposeQuaternion');
      mask Display: disp('q''');
  vB : Outport
  wires:
  Product/1 -> vB/1
  quat product1/1(q1*q2) -> Demux/1
  quat product/1(q1*q2) -> quat product1/1(q1)
  Mux/1 -> quat product/2(q2)
  transposeQuaternion/1(q') -> quat product/1(q1)
  qA2B/1 -> quat product1/2(q2), transposeQuaternion/1(q)
  vA/1 -> Mux/2
  Constant/1 -> Mux/1
  Demux/1 -> Product/1
  Demux/2 -> Product/2

== system attitude3d/Subsystem2/frame change9 ==
  vA : Inport
  qA2B : Inport  Port=2
  Constant : Constant
  Demux : Demux  Outputs=[1 3]
  Mux : Mux  Inputs=2
  Product : Product  Inputs=/*  SaturateOnIntegerOverflow=on  OutDataTypeStr=Inherit: Same as first input
  quat product : Subsystem
      mask Display:
      | plot(0.5+cos(linspace(0,2*pi,65))*0.3,0.5+sin(linspace(0,2*pi,65))*0.3);
      | plot([.29 .71],[.29 .71]);
      | plot([.71 .29],[.29 .71]);
  quat product1 : Subsystem
      mask Display:
      | plot(0.5+cos(linspace(0,2*pi,65))*0.3,0.5+sin(linspace(0,2*pi,65))*0.3);
      | plot([.29 .71],[.29 .71]);
      | plot([.71 .29],[.29 .71]);
  transposeQuaternion : Subsystem  mask(transposeQuaternion){}
      mask help:
      | Compute the transpose (inverse or conjugate) of the input quaternion
      |
      | Inputs:
      |   q     Quaternion
      |
      | Outputs:
      |   qt     Transpose of the input quaternion
      mask Help: eval('starDoc simulink/transposeQuaternion');
      mask Display: disp('q''');
  vB : Outport
  wires:
  Product/1 -> vB/1
  quat product1/1(q1*q2) -> Demux/1
  quat product/1(q1*q2) -> quat product1/1(q1)
  Mux/1 -> quat product/2(q2)
  transposeQuaternion/1(q') -> quat product/1(q1)
  qA2B/1 -> quat product1/2(q2), transposeQuaternion/1(q)
  vA/1 -> Mux/2
  Constant/1 -> Mux/1
  Demux/1 -> Product/1
  Demux/2 -> Product/2

== system attitude3d/Quaternion Propagator/qDot/quat product ==
  q1 : Inport
  q2 : Inport  Port=2
  Cross Product : Subsystem  Tag=68  mask(CrossProduct){}
      mask help: Compute the cross product of two 3-vectors : y = u1 x u2
      mask Display:
      | plot([.4 .6],[.4 .6]);
      | plot([.6 .4],[.4 .6]);
  Demux : Demux  Outputs=[1 3]
  Demux1 : Demux  Outputs=[1 3]
  Dot Product : DotProduct  InputSameDT=on  OutDataTypeStr=Inherit: Inherit via internal rule
  Mux : Mux  Inputs=2
  Product : Product  SaturateOnIntegerOverflow=on  OutDataTypeStr=Inherit: Same as first input
  Product1 : Product  SaturateOnIntegerOverflow=on  OutDataTypeStr=Inherit: Same as first input
  Product2 : Product  SaturateOnIntegerOverflow=on  OutDataTypeStr=Inherit: Same as first input
  Sum : Sum  Inputs=+++  SaturateOnIntegerOverflow=on
  Sum1 : Sum  Inputs=|+-  SaturateOnIntegerOverflow=on
  q1*q2 : Outport
  wires:
  q2/1 -> Demux1/1
  Mux/1 -> q1*q2/1
  q1/1 -> Demux/1
  Sum1/1 -> Mux/1  "scalar"
  Dot Product/1 -> Sum1/2
  Product2/1 -> Sum1/1
  Sum/1 -> Mux/2  "vector"
  Product1/1 -> Sum/3
  Product/1 -> Sum/1
  Cross Product/1(u1xu2) -> Sum/2
  Demux1/2 -> Dot Product/1, Product/2, Cross Product/2(u2)
  Demux1/1 -> Product2/2, Product1/1
  Demux/1 -> Product2/1, Product/1
  Demux/2 -> Dot Product/2, Cross Product/1(u1), Product1/2

== system attitude3d/Subsystem2/frame change5/quat product ==
  q1 : Inport
  q2 : Inport  Port=2
  Cross Product : Subsystem  Tag=68  mask(CrossProduct){}
      mask help: Compute the cross product of two 3-vectors : y = u1 x u2
      mask Display:
      | plot([.4 .6],[.4 .6]);
      | plot([.6 .4],[.4 .6]);
  Demux : Demux  Outputs=[1 3]
  Demux1 : Demux  Outputs=[1 3]
  Dot Product : DotProduct  InputSameDT=on  OutDataTypeStr=Inherit: Inherit via internal rule
  Mux : Mux  Inputs=2
  Product : Product  SaturateOnIntegerOverflow=on  OutDataTypeStr=Inherit: Same as first input
  Product1 : Product  SaturateOnIntegerOverflow=on  OutDataTypeStr=Inherit: Same as first input
  Product2 : Product  SaturateOnIntegerOverflow=on  OutDataTypeStr=Inherit: Same as first input
  Sum : Sum  Inputs=+++  SaturateOnIntegerOverflow=on
  Sum1 : Sum  Inputs=|+-  SaturateOnIntegerOverflow=on
  q1*q2 : Outport
  wires:
  Demux/2 -> Product1/2, Cross Product/1(u1), Dot Product/2
  Demux/1 -> Product/1, Product2/1
  Demux1/1 -> Product1/1, Product2/2
  Demux1/2 -> Cross Product/2(u2), Product/2, Dot Product/1
  Cross Product/1(u1xu2) -> Sum/2
  Product/1 -> Sum/1
  Product1/1 -> Sum/3
  Sum/1 -> Mux/2  "vector"
  Product2/1 -> Sum1/1
  Dot Product/1 -> Sum1/2
  Sum1/1 -> Mux/1  "scalar"
  q1/1 -> Demux/1
  Mux/1 -> q1*q2/1
  q2/1 -> Demux1/1

== system attitude3d/Subsystem2/frame change5/quat product1 ==
  q1 : Inport
  q2 : Inport  Port=2
  Cross Product : Subsystem  Tag=68  mask(CrossProduct){}
      mask help: Compute the cross product of two 3-vectors : y = u1 x u2
      mask Display:
      | plot([.4 .6],[.4 .6]);
      | plot([.6 .4],[.4 .6]);
  Demux : Demux  Outputs=[1 3]
  Demux1 : Demux  Outputs=[1 3]
  Dot Product : DotProduct  InputSameDT=on  OutDataTypeStr=Inherit: Inherit via internal rule
  Mux : Mux  Inputs=2
  Product : Product  SaturateOnIntegerOverflow=on  OutDataTypeStr=Inherit: Same as first input
  Product1 : Product  SaturateOnIntegerOverflow=on  OutDataTypeStr=Inherit: Same as first input
  Product2 : Product  SaturateOnIntegerOverflow=on  OutDataTypeStr=Inherit: Same as first input
  Sum : Sum  Inputs=+++  SaturateOnIntegerOverflow=on
  Sum1 : Sum  Inputs=|+-  SaturateOnIntegerOverflow=on
  q1*q2 : Outport
  wires:
  q2/1 -> Demux1/1
  Mux/1 -> q1*q2/1
  q1/1 -> Demux/1
  Sum1/1 -> Mux/1  "scalar"
  Dot Product/1 -> Sum1/2
  Product2/1 -> Sum1/1
  Sum/1 -> Mux/2  "vector"
  Product1/1 -> Sum/3
  Product/1 -> Sum/1
  Cross Product/1(u1xu2) -> Sum/2
  Demux1/2 -> Dot Product/1, Product/2, Cross Product/2(u2)
  Demux1/1 -> Product2/2, Product1/1
  Demux/1 -> Product2/1, Product/1
  Demux/2 -> Dot Product/2, Cross Product/1(u1), Product1/2

== system attitude3d/Subsystem2/frame change5/transposeQuaternion ==
  q : Inport
  Gain1 : Gain  Gain=[1 -1 -1 -1]  SaturateOnIntegerOverflow=on  OutDataTypeStr=Inherit: Same as input  ParamDataTypeStr=Inherit: Same as input
  q' : Outport
  wires:
  q/1 -> Gain1/1
  Gain1/1 -> q'/1

== system attitude3d/Subsystem2/frame change6/quat product ==
  q1 : Inport
  q2 : Inport  Port=2
  Cross Product : Subsystem  Tag=68  mask(CrossProduct){}
      mask help: Compute the cross product of two 3-vectors : y = u1 x u2
      mask Display:
      | plot([.4 .6],[.4 .6]);
      | plot([.6 .4],[.4 .6]);
  Demux : Demux  Outputs=[1 3]
  Demux1 : Demux  Outputs=[1 3]
  Dot Product : DotProduct  InputSameDT=on  OutDataTypeStr=Inherit: Inherit via internal rule
  Mux : Mux  Inputs=2
  Product : Product  SaturateOnIntegerOverflow=on  OutDataTypeStr=Inherit: Same as first input
  Product1 : Product  SaturateOnIntegerOverflow=on  OutDataTypeStr=Inherit: Same as first input
  Product2 : Product  SaturateOnIntegerOverflow=on  OutDataTypeStr=Inherit: Same as first input
  Sum : Sum  Inputs=+++  SaturateOnIntegerOverflow=on
  Sum1 : Sum  Inputs=|+-  SaturateOnIntegerOverflow=on
  q1*q2 : Outport
  wires:
  Demux/2 -> Product1/2, Cross Product/1(u1), Dot Product/2
  Demux/1 -> Product/1, Product2/1
  Demux1/1 -> Product1/1, Product2/2
  Demux1/2 -> Cross Product/2(u2), Product/2, Dot Product/1
  Cross Product/1(u1xu2) -> Sum/2
  Product/1 -> Sum/1
  Product1/1 -> Sum/3
  Sum/1 -> Mux/2  "vector"
  Product2/1 -> Sum1/1
  Dot Product/1 -> Sum1/2
  Sum1/1 -> Mux/1  "scalar"
  q1/1 -> Demux/1
  Mux/1 -> q1*q2/1
  q2/1 -> Demux1/1

== system attitude3d/Subsystem2/frame change6/quat product1 ==
  q1 : Inport
  q2 : Inport  Port=2
  Cross Product : Subsystem  Tag=68  mask(CrossProduct){}
      mask help: Compute the cross product of two 3-vectors : y = u1 x u2
      mask Display:
      | plot([.4 .6],[.4 .6]);
      | plot([.6 .4],[.4 .6]);
  Demux : Demux  Outputs=[1 3]
  Demux1 : Demux  Outputs=[1 3]
  Dot Product : DotProduct  InputSameDT=on  OutDataTypeStr=Inherit: Inherit via internal rule
  Mux : Mux  Inputs=2
  Product : Product  SaturateOnIntegerOverflow=on  OutDataTypeStr=Inherit: Same as first input
  Product1 : Product  SaturateOnIntegerOverflow=on  OutDataTypeStr=Inherit: Same as first input
  Product2 : Product  SaturateOnIntegerOverflow=on  OutDataTypeStr=Inherit: Same as first input
  Sum : Sum  Inputs=+++  SaturateOnIntegerOverflow=on
  Sum1 : Sum  Inputs=|+-  SaturateOnIntegerOverflow=on
  q1*q2 : Outport
  wires:
  q2/1 -> Demux1/1
  Mux/1 -> q1*q2/1
  q1/1 -> Demux/1
  Sum1/1 -> Mux/1  "scalar"
  Dot Product/1 -> Sum1/2
  Product2/1 -> Sum1/1
  Sum/1 -> Mux/2  "vector"
  Product1/1 -> Sum/3
  Product/1 -> Sum/1
  Cross Product/1(u1xu2) -> Sum/2
  Demux1/2 -> Dot Product/1, Product/2, Cross Product/2(u2)
  Demux1/1 -> Product2/2, Product1/1
  Demux/1 -> Product2/1, Product/1
  Demux/2 -> Dot Product/2, Cross Product/1(u1), Product1/2

== system attitude3d/Subsystem2/frame change6/transposeQuaternion ==
  q : Inport
  Gain1 : Gain  Gain=[1 -1 -1 -1]  SaturateOnIntegerOverflow=on  OutDataTypeStr=Inherit: Same as input  ParamDataTypeStr=Inherit: Same as input
  q' : Outport
  wires:
  q/1 -> Gain1/1
  Gain1/1 -> q'/1

== system attitude3d/Subsystem2/frame change7/quat product ==
  q1 : Inport
  q2 : Inport  Port=2
  Cross Product : Subsystem  Tag=68  mask(CrossProduct){}
      mask help: Compute the cross product of two 3-vectors : y = u1 x u2
      mask Display:
      | plot([.4 .6],[.4 .6]);
      | plot([.6 .4],[.4 .6]);
  Demux : Demux  Outputs=[1 3]
  Demux1 : Demux  Outputs=[1 3]
  Dot Product : DotProduct  InputSameDT=on  OutDataTypeStr=Inherit: Inherit via internal rule
  Mux : Mux  Inputs=2
  Product : Product  SaturateOnIntegerOverflow=on  OutDataTypeStr=Inherit: Same as first input
  Product1 : Product  SaturateOnIntegerOverflow=on  OutDataTypeStr=Inherit: Same as first input
  Product2 : Product  SaturateOnIntegerOverflow=on  OutDataTypeStr=Inherit: Same as first input
  Sum : Sum  Inputs=+++  SaturateOnIntegerOverflow=on
  Sum1 : Sum  Inputs=|+-  SaturateOnIntegerOverflow=on
  q1*q2 : Outport
  wires:
  Demux/2 -> Product1/2, Cross Product/1(u1), Dot Product/2
  Demux/1 -> Product/1, Product2/1
  Demux1/1 -> Product1/1, Product2/2
  Demux1/2 -> Cross Product/2(u2), Product/2, Dot Product/1
  Cross Product/1(u1xu2) -> Sum/2
  Product/1 -> Sum/1
  Product1/1 -> Sum/3
  Sum/1 -> Mux/2  "vector"
  Product2/1 -> Sum1/1
  Dot Product/1 -> Sum1/2
  Sum1/1 -> Mux/1  "scalar"
  q1/1 -> Demux/1
  Mux/1 -> q1*q2/1
  q2/1 -> Demux1/1

== system attitude3d/Subsystem2/frame change7/quat product1 ==
  q1 : Inport
  q2 : Inport  Port=2
  Cross Product : Subsystem  Tag=68  mask(CrossProduct){}
      mask help: Compute the cross product of two 3-vectors : y = u1 x u2
      mask Display:
      | plot([.4 .6],[.4 .6]);
      | plot([.6 .4],[.4 .6]);
  Demux : Demux  Outputs=[1 3]
  Demux1 : Demux  Outputs=[1 3]
  Dot Product : DotProduct  InputSameDT=on  OutDataTypeStr=Inherit: Inherit via internal rule
  Mux : Mux  Inputs=2
  Product : Product  SaturateOnIntegerOverflow=on  OutDataTypeStr=Inherit: Same as first input
  Product1 : Product  SaturateOnIntegerOverflow=on  OutDataTypeStr=Inherit: Same as first input
  Product2 : Product  SaturateOnIntegerOverflow=on  OutDataTypeStr=Inherit: Same as first input
  Sum : Sum  Inputs=+++  SaturateOnIntegerOverflow=on
  Sum1 : Sum  Inputs=|+-  SaturateOnIntegerOverflow=on
  q1*q2 : Outport
  wires:
  q2/1 -> Demux1/1
  Mux/1 -> q1*q2/1
  q1/1 -> Demux/1
  Sum1/1 -> Mux/1  "scalar"
  Dot Product/1 -> Sum1/2
  Product2/1 -> Sum1/1
  Sum/1 -> Mux/2  "vector"
  Product1/1 -> Sum/3
  Product/1 -> Sum/1
  Cross Product/1(u1xu2) -> Sum/2
  Demux1/2 -> Dot Product/1, Product/2, Cross Product/2(u2)
  Demux1/1 -> Product2/2, Product1/1
  Demux/1 -> Product2/1, Product/1
  Demux/2 -> Dot Product/2, Cross Product/1(u1), Product1/2

== system attitude3d/Subsystem2/frame change7/transposeQuaternion ==
  q : Inport
  Gain1 : Gain  Gain=[1 -1 -1 -1]  SaturateOnIntegerOverflow=on  OutDataTypeStr=Inherit: Same as input  ParamDataTypeStr=Inherit: Same as input
  q' : Outport
  wires:
  q/1 -> Gain1/1
  Gain1/1 -> q'/1

== system attitude3d/Subsystem2/frame change8/quat product ==
  q1 : Inport
  q2 : Inport  Port=2
  Cross Product : Subsystem  Tag=68  mask(CrossProduct){}
      mask help: Compute the cross product of two 3-vectors : y = u1 x u2
      mask Display:
      | plot([.4 .6],[.4 .6]);
      | plot([.6 .4],[.4 .6]);
  Demux : Demux  Outputs=[1 3]
  Demux1 : Demux  Outputs=[1 3]
  Dot Product : DotProduct  InputSameDT=on  OutDataTypeStr=Inherit: Inherit via internal rule
  Mux : Mux  Inputs=2
  Product : Product  SaturateOnIntegerOverflow=on  OutDataTypeStr=Inherit: Same as first input
  Product1 : Product  SaturateOnIntegerOverflow=on  OutDataTypeStr=Inherit: Same as first input
  Product2 : Product  SaturateOnIntegerOverflow=on  OutDataTypeStr=Inherit: Same as first input
  Sum : Sum  Inputs=+++  SaturateOnIntegerOverflow=on
  Sum1 : Sum  Inputs=|+-  SaturateOnIntegerOverflow=on
  q1*q2 : Outport
  wires:
  Demux/2 -> Product1/2, Cross Product/1(u1), Dot Product/2
  Demux/1 -> Product/1, Product2/1
  Demux1/1 -> Product1/1, Product2/2
  Demux1/2 -> Cross Product/2(u2), Product/2, Dot Product/1
  Cross Product/1(u1xu2) -> Sum/2
  Product/1 -> Sum/1
  Product1/1 -> Sum/3
  Sum/1 -> Mux/2  "vector"
  Product2/1 -> Sum1/1
  Dot Product/1 -> Sum1/2
  Sum1/1 -> Mux/1  "scalar"
  q1/1 -> Demux/1
  Mux/1 -> q1*q2/1
  q2/1 -> Demux1/1

== system attitude3d/Subsystem2/frame change8/quat product1 ==
  q1 : Inport
  q2 : Inport  Port=2
  Cross Product : Subsystem  Tag=68  mask(CrossProduct){}
      mask help: Compute the cross product of two 3-vectors : y = u1 x u2
      mask Display:
      | plot([.4 .6],[.4 .6]);
      | plot([.6 .4],[.4 .6]);
  Demux : Demux  Outputs=[1 3]
  Demux1 : Demux  Outputs=[1 3]
  Dot Product : DotProduct  InputSameDT=on  OutDataTypeStr=Inherit: Inherit via internal rule
  Mux : Mux  Inputs=2
  Product : Product  SaturateOnIntegerOverflow=on  OutDataTypeStr=Inherit: Same as first input
  Product1 : Product  SaturateOnIntegerOverflow=on  OutDataTypeStr=Inherit: Same as first input
  Product2 : Product  SaturateOnIntegerOverflow=on  OutDataTypeStr=Inherit: Same as first input
  Sum : Sum  Inputs=+++  SaturateOnIntegerOverflow=on
  Sum1 : Sum  Inputs=|+-  SaturateOnIntegerOverflow=on
  q1*q2 : Outport
  wires:
  q2/1 -> Demux1/1
  Mux/1 -> q1*q2/1
  q1/1 -> Demux/1
  Sum1/1 -> Mux/1  "scalar"
  Dot Product/1 -> Sum1/2
  Product2/1 -> Sum1/1
  Sum/1 -> Mux/2  "vector"
  Product1/1 -> Sum/3
  Product/1 -> Sum/1
  Cross Product/1(u1xu2) -> Sum/2
  Demux1/2 -> Dot Product/1, Product/2, Cross Product/2(u2)
  Demux1/1 -> Product2/2, Product1/1
  Demux/1 -> Product2/1, Product/1
  Demux/2 -> Dot Product/2, Cross Product/1(u1), Product1/2

== system attitude3d/Subsystem2/frame change8/transposeQuaternion ==
  q : Inport
  Gain1 : Gain  Gain=[1 -1 -1 -1]  SaturateOnIntegerOverflow=on  OutDataTypeStr=Inherit: Same as input  ParamDataTypeStr=Inherit: Same as input
  q' : Outport
  wires:
  q/1 -> Gain1/1
  Gain1/1 -> q'/1

== system attitude3d/Subsystem2/frame change9/quat product ==
  q1 : Inport
  q2 : Inport  Port=2
  Cross Product : Subsystem  Tag=68  mask(CrossProduct){}
      mask help: Compute the cross product of two 3-vectors : y = u1 x u2
      mask Display:
      | plot([.4 .6],[.4 .6]);
      | plot([.6 .4],[.4 .6]);
  Demux : Demux  Outputs=[1 3]
  Demux1 : Demux  Outputs=[1 3]
  Dot Product : DotProduct  InputSameDT=on  OutDataTypeStr=Inherit: Inherit via internal rule
  Mux : Mux  Inputs=2
  Product : Product  SaturateOnIntegerOverflow=on  OutDataTypeStr=Inherit: Same as first input
  Product1 : Product  SaturateOnIntegerOverflow=on  OutDataTypeStr=Inherit: Same as first input
  Product2 : Product  SaturateOnIntegerOverflow=on  OutDataTypeStr=Inherit: Same as first input
  Sum : Sum  Inputs=+++  SaturateOnIntegerOverflow=on
  Sum1 : Sum  Inputs=|+-  SaturateOnIntegerOverflow=on
  q1*q2 : Outport
  wires:
  Demux/2 -> Product1/2, Cross Product/1(u1), Dot Product/2
  Demux/1 -> Product/1, Product2/1
  Demux1/1 -> Product1/1, Product2/2
  Demux1/2 -> Cross Product/2(u2), Product/2, Dot Product/1
  Cross Product/1(u1xu2) -> Sum/2
  Product/1 -> Sum/1
  Product1/1 -> Sum/3
  Sum/1 -> Mux/2  "vector"
  Product2/1 -> Sum1/1
  Dot Product/1 -> Sum1/2
  Sum1/1 -> Mux/1  "scalar"
  q1/1 -> Demux/1
  Mux/1 -> q1*q2/1
  q2/1 -> Demux1/1

== system attitude3d/Subsystem2/frame change9/quat product1 ==
  q1 : Inport
  q2 : Inport  Port=2
  Cross Product : Subsystem  Tag=68  mask(CrossProduct){}
      mask help: Compute the cross product of two 3-vectors : y = u1 x u2
      mask Display:
      | plot([.4 .6],[.4 .6]);
      | plot([.6 .4],[.4 .6]);
  Demux : Demux  Outputs=[1 3]
  Demux1 : Demux  Outputs=[1 3]
  Dot Product : DotProduct  InputSameDT=on  OutDataTypeStr=Inherit: Inherit via internal rule
  Mux : Mux  Inputs=2
  Product : Product  SaturateOnIntegerOverflow=on  OutDataTypeStr=Inherit: Same as first input
  Product1 : Product  SaturateOnIntegerOverflow=on  OutDataTypeStr=Inherit: Same as first input
  Product2 : Product  SaturateOnIntegerOverflow=on  OutDataTypeStr=Inherit: Same as first input
  Sum : Sum  Inputs=+++  SaturateOnIntegerOverflow=on
  Sum1 : Sum  Inputs=|+-  SaturateOnIntegerOverflow=on
  q1*q2 : Outport
  wires:
  q2/1 -> Demux1/1
  Mux/1 -> q1*q2/1
  q1/1 -> Demux/1
  Sum1/1 -> Mux/1  "scalar"
  Dot Product/1 -> Sum1/2
  Product2/1 -> Sum1/1
  Sum/1 -> Mux/2  "vector"
  Product1/1 -> Sum/3
  Product/1 -> Sum/1
  Cross Product/1(u1xu2) -> Sum/2
  Demux1/2 -> Dot Product/1, Product/2, Cross Product/2(u2)
  Demux1/1 -> Product2/2, Product1/1
  Demux/1 -> Product2/1, Product/1
  Demux/2 -> Dot Product/2, Cross Product/1(u1), Product1/2
